simulink model "block_test"  (R2013a)
settings: Solver=ode45  StartTime=0.0  StopTime=10.0  RelTol=1e-3
settings Model: Creator=mainster  LastModifiedBy=mainster

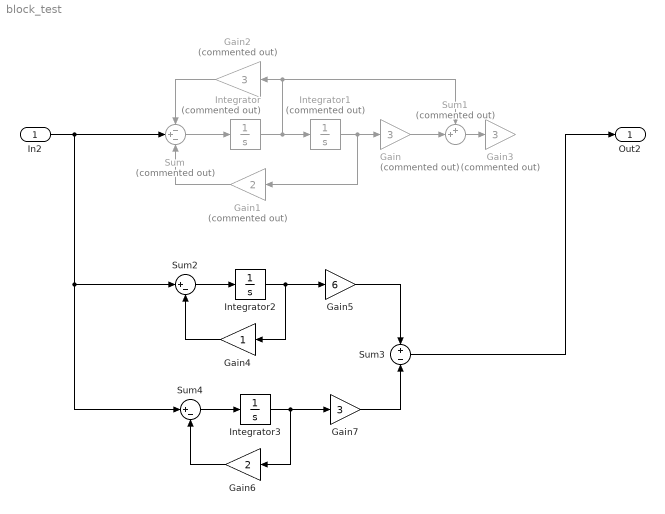
== system block_test ==
  In2 : Inport
  Gain : Gain  Commented=on  Gain=3
  Gain1 : Gain  Commented=on  Gain=2
  Gain2 : Gain  Commented=on  Gain=3
  Gain3 : Gain  Commented=on  Gain=3
  Gain4 : Gain
  Gain5 : Gain  Gain=6
  Gain6 : Gain  Gain=2
  Gain7 : Gain  Gain=3
  Integrator : Integrator  Commented=on
  Integrator1 : Integrator  Commented=on
  Integrator2 : Integrator
  Integrator3 : Integrator
  Sum : Sum  Commented=on  Inputs=-+-
  Sum1 : Sum  Commented=on  Inputs=++|
  Sum2 : Sum  Inputs=|+-
  Sum3 : Sum  Inputs=+|-
  Sum4 : Sum  Inputs=|+-
  Out2 : Outport
  wires:
  Gain2/1 -> Sum/1
  Gain1/1 -> Sum/3
  Sum/1 -> Integrator/1
  Integrator/1 -> Sum1/1, Gain2/1, Integrator1/1
  Integrator1/1 -> Gain1/1, Gain/1
  Gain/1 -> Sum1/2
  Sum1/1 -> Gain3/1
  Sum2/1 -> Integrator2/1
  Integrator2/1 -> Gain5/1, Gain4/1
  In2/1 -> Sum4/1, Sum2/1, Sum/2
  Gain4/1 -> Sum2/2
  Gain5/1 -> Sum3/1
  Sum4/1 -> Integrator3/1
  Integrator3/1 -> Gain7/1, Gain6/1
  Gain6/1 -> Sum4/2
  Gain7/1 -> Sum3/2
  Sum3/1 -> Out2/1
